simulink model "Modello_corretto_with_observer"  (R2023b)
settings: Solver=VariableStepAuto  StartTime=0.0  StopTime=Tend_slk  RelTol=1e-3
undefined symbols (not defined in the file): Alin, Blin, Clin, Dlin, L, param, Ts_slk, x0
settings Model: Creator=asus  LastModifiedBy=asus
settings OptimizationCC: ReuseModelBlockBuffer=off
settings DebuggingCC: SignalInfNanChecking=error

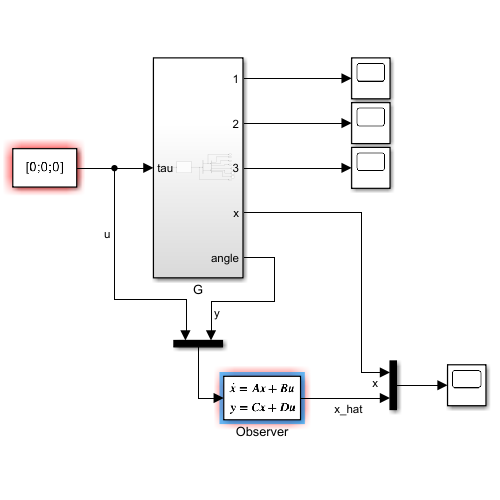
[thumbnail: Simulink's stored preview of the top-level diagram]
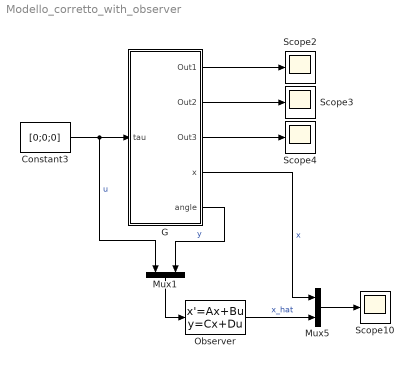
== system Modello_corretto_with_observer ==
  Constant3 : Constant  Value=[0;0;0]  VectorParams1D=off  SampleTime=Ts_slk
  G : Subsystem
  Mux1 : Mux  Inputs=2
  Mux5 : Mux  Inputs=2
  Observer : StateSpace  A=Alin-L*Clin  B=[Blin-L*Dlin L]  C=eye(6)  D=zeros(6,6)  InitialCondition=0
  Scope{2..4,10} (4 alike) : Scope
  wires:
  G/1(Out1) -> Scope2/1
  G/2(Out2) -> Scope3/1
  G/3(Out3) -> Scope4/1
  G/4(x) -> Mux5/1  "x"
  Mux5/1 -> Scope10/1
  Observer/1 -> Mux5/2  "x_hat"
  G/5(angle) -> Mux1/2  "y"
  Mux1/1 -> Observer/1
  Constant3/1 -> Mux1/1, G/1("tau ")  "u"

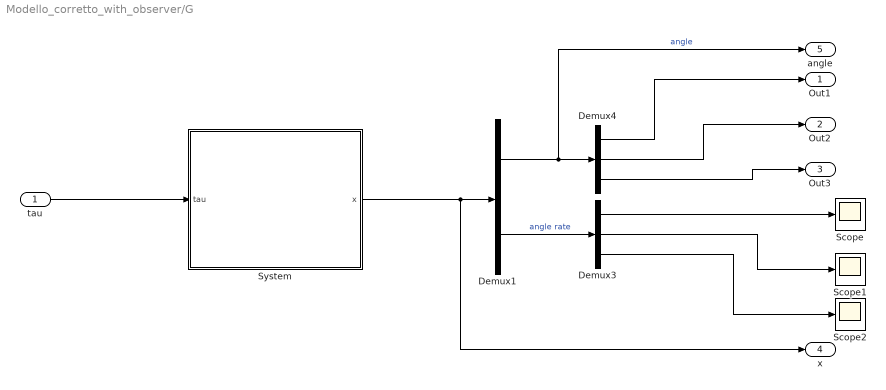
== system Modello_corretto_with_observer/G ==
  "tau " : Inport
  Demux1 : Demux  Outputs=2
  Demux3 : Demux  Outputs=3
  Demux4 : Demux  Outputs=3
  Scope : Scope
  Scope1 : Scope
  Scope2 : Scope
  System : Subsystem
  Out1 : Outport
  Out2 : Outport  Port=2
  Out3 : Outport  Port=3
  x : Outport  Port=4
  angle : Outport  Port=5
  wires:
  Demux4/3 -> Out3/1
  System/1(x) -> x/1, Demux1/1
  Demux3/1 -> Scope/1
  Demux4/1 -> Out1/1
  Demux1/1 -> angle/1, Demux4/1  "angle"
  Demux1/2 -> Demux3/1  "angle rate"
  Demux3/2 -> Scope1/1
  Demux4/2 -> Out2/1
  "tau "/1 -> System/1("tau ")
  Demux3/3 -> Scope2/1

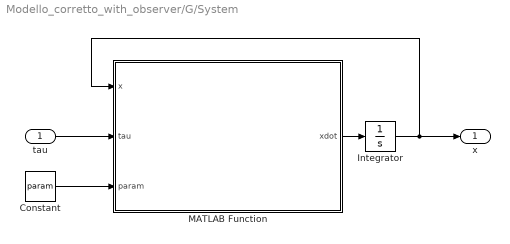
== system Modello_corretto_with_observer/G/System ==
  "tau " : Inport
  Constant : Constant  Value=param
  Integrator : Integrator  InitialCondition=x0
  MATLAB Function : MATLAB Function  TreatAsAtomicUnit=on
  x : Outport
  wires:
  Integrator/1 -> MATLAB Function/1(x), x/1
  MATLAB Function/1(xdot) -> Integrator/1
  "tau "/1 -> MATLAB Function/2(tau)
  Constant/1 -> MATLAB Function/3(param)

== matlab function Modello_corretto_with_observer/G/System/MATLAB Function ==
  data: x input; tau input; xdot output; param input
function xdot =quadcopter(x,tau,param)
% Inputs:
%           x       (model state)
%           tau     (torque)           
%           param   (model parameters)
%
% Outputs:  x_dot  (derivative of the state with respect to time)

% Parameters
g        =       9.81;           %  gravity acceleration (m/s^2)
Ixx      =       param(1,1);     %  moment of inertia 
Iyy      =       param(2,1);     %  moment of inertia
Izz      =       param(3,1);     %  moment of inertia 

% States
phi      =       x(1,1);     %  roll angle (rad)
theta    =       x(2,1);     %  pitch angle (rad)
psi      =       x(3,1);     %  yaw angle (rad)  
phi_dot  =       x(4,1);     %  roll rate (rad/s)
theta_dot=       x(5,1);     %  pitch rate (rad/s)
psi_dot  =       x(6,1);     %  yaw rate (rad/s)  

cph         =       cos(phi);
cth         =       cos(theta);
cps         =       cos(psi);
sph         =       sin(phi);
sth         =       sin(theta);
sps         =       sin(psi);

% torques
tau_1    =       tau(1,1);   %  roll torque 
tau_2    =       tau(2,1);   %  pitch torque 
tau_3    =       tau(3,1);   %  yaw torque   

% Coriolis matrix
C11=  0;
C12= (Iyy-Izz)*(theta_dot*cph*sph+psi_dot*sph^2*cth)+(Izz-Iyy)*psi_dot*cph^2*cth-Ixx*psi_dot*cth;
C13= (Izz-Iyy)*psi_dot*cph*sph*cth^2;
C21= (Izz-Iyy)*(theta_dot*cph*sph+psi_dot*sph*cth)+(Iyy-Izz)*psi_dot*cph^2*cth+Ixx*psi_dot*cth;
C22= (Izz-Iyy)*psi_dot*cph*sph;
C23= -Ixx*psi_dot*sth*cth+Iyy*psi_dot*sph^2*sth*cth+Izz*psi_dot*cph^2*sth*cth;
C31= (Iyy-Izz)*psi_dot*cth^2*sph*cph-Ixx*theta_dot*cth;
C32= (Izz-Iyy)*(theta_dot*cph*sph*sth+phi_dot*sph^2*cth)+(Iyy-Izz)*phi_dot*cph^2*cth+Ixx*psi_dot*sth*cth-Iyy*psi_dot*sph^2*sth*cth-Izz*psi_dot*cph^2*sth*cth;
C33= (Iyy-Izz)*phi_dot*cph*sph*cth^2-Iyy*theta_dot*sph^2*cth*sth-Izz*theta_dot*cph^2*cth*sth+Ixx*theta_dot*cth*sth;

C  = [C11 C12 C13;
    C21 C22 C23;
    C31 C32 C33];

% Inertia matrix
J11= Ixx;
J12= 0;
J13= -Ixx*sth;
J21= 0;
J22= Iyy*cph^2+Izz*sph^2;
J23= (Iyy-Izz)*cph*sph*cth;
J31= -Ixx*sth;
J32= (Iyy-Izz)*cph*sph*cth;
J33= Ixx*sth^2+Iyy*sph^2*cth^2+Izz*cph^2*cth^2;

J  = [J11 J12 J13;
    J21 J22 J23;
    J31 J32 J33];

%% Model Equation 
invJ = [ (J22*J33 - J23*J32)/(J11*J22*J33 - J11*J23*J32 - J12*J21*J33 + J12*J23*J31 + J13*J21*J32 - J13*J22*J31), -(J12*J33 - J13*J32)/(J11*J22*J33 - J11*J23*J32 - J12*J21*J33 + J12*J23*J31 + J13*J21*J32 - J13*J22*J31),  (J12*J23 - J13*J22)/(J11*J22*J33 - J11*J23*J32 - J12*J21*J33 + J12*J23*J31 + J13*J21*J32 - J13*J22*J31);
         -(J21*J33 - J23*J31)/(J11*J22*J33 - J11*J23*J32 - J12*J21*J33 + J12*J23*J31 + J13*J21*J32 - J13*J22*J31),  (J11*J33 - J13*J31)/(J11*J22*J33 - J11*J23*J32 - J12*J21*J33 + J12*J23*J31 + J13*J21*J32 - J13*J22*J31), -(J11*J23 - J13*J21)/(J11*J22*J33 - J11*J23*J32 - J12*J21*J33 + J12*J23*J31 + J13*J21*J32 - J13*J22*J31);
         (J21*J32 - J22*J31)/(J11*J22*J33 - J11*J23*J32 - J12*J21*J33 + J12*J23*J31 + J13*J21*J32 - J13*J22*J31), -(J11*J32 - J12*J31)/(J11*J22*J33 - J11*J23*J32 - J12*J21*J33 + J12*J23*J31 + J13*J21*J32 - J13*J22*J31),  (J11*J22 - J12*J21)/(J11*J22*J33 - J11*J23*J32 - J12*J21*J33 + J12*J23*J31 + J13*J21*J32 - J13*J22*J31);];

xdot        = zeros(6,1);
xdot(1:3,1) = x(4:6,1);
xdot(4:6,1) = invJ*(tau - C*x(4:6,1));
